simulink model "VsourceInverterZsourceRectifier"  (R2017b)
settings: Solver=ode45  StartTime=0.0  StopTime=0.05  RelTol=1e-3  EnableMultiTasking=on
InitFcn:
  | Fs=100e3;
  | w=Fs*2*pi;
  | 
  | Vdc=100;
  | 
  | LP=200e-6;
  | LS=LP;
  | 
  | CP=1/w^2/LP;
  | CS=1/w^2/LS;
  | 
  | MPS=20e-6;
  | 
  | 
  | Rlp=0.1;
  | Rls=0.1;
libraries: powerlib x30, powerlib_meascontrol x8, simulink x2
settings Model: Creator=User  LastModifiedBy=SuperWindows
settings DataIOCC: FinalStateName=xInitial  LimitDataPoints=on  SaveFinalState=on  SaveFormat=Array
settings OptimizationCC: LifeSpan=inf
settings DebuggingCC: SolverPrmCheckMsg=warning  SFUnexpectedBacktrackingDiag=warning  SFNoUnconditionalDefaultTransitionDiag=warning  SFExecutionAtInitializationDiag=none
settings HardwareCC: ProdBitPerPointer=32  ProdBitPerSizeT=32  ProdBitPerPtrDiffT=32  ProdLargestAtomicFloat=None  ProdIntDivRoundTo=Undefined  ProdEndianess=Unspecified  ProdWordSize=32  ProdHWDeviceType=32-bit Generic
settings ModelReferenceCC: PropagateSignalLabelsOutOfModel=off
settings CodeAppCC: StateflowObjectComments=on
settings GRTTargetCC: TargetLangStandard=C89/C90 (ANSI)  GeneratePreprocessorConditionals=Disable all
settings ConfigComp: CovMetricSettings=dw  CovHtmlReporting=on  CovSaveCumulativeToWorkspaceVar=on  CovSaveSingleToWorkspaceVar=on  CovExternalEMLEnable=off  CovSFcnEnable=off
settings SimscapeCC: SimscapeNormalizeSystem=off

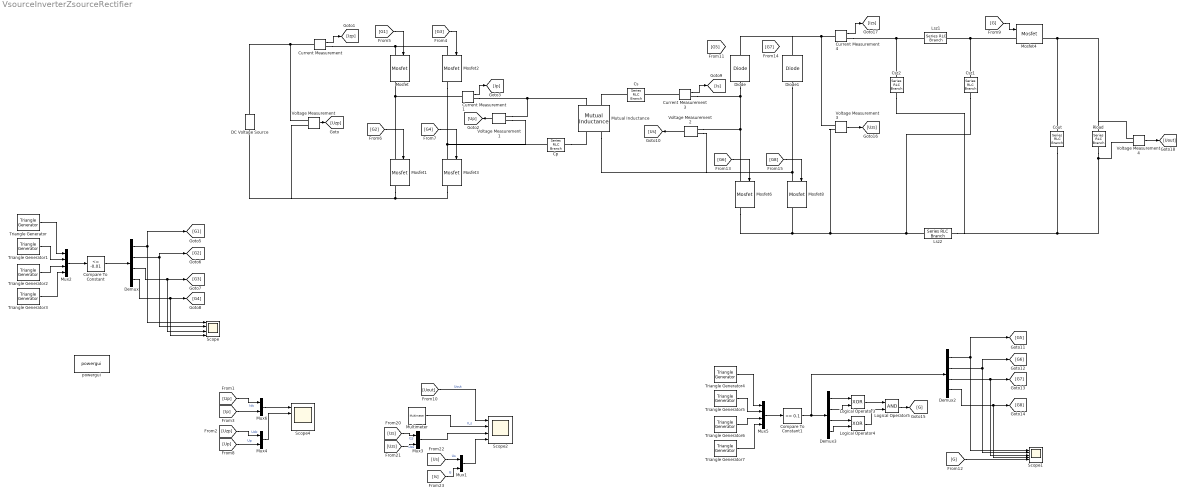
== system VsourceInverterZsourceRectifier ==
  Compare To Constant : simulink/Logic and Bit Operations/Compare To Constant  relop=<=  const=-0.01  OutDataTypeStr=boolean
  Compare To Constant1 : simulink/Logic and Bit Operations/Compare To Constant  relop=<=  const=0.1  OutDataTypeStr=boolean
  Cout : powerlib/Elements/Series RLC Branch  LConnTagsString=__new0  RConnTagsString=__new0  BranchType=C  Resistance=1  Inductance=1e-3  SetiL0=off  InitialCurrent=0  Capacitance=470e-6  Setx0=off  InitialVoltage=100  Measurements=Branch voltage and current
  Cp : powerlib/Elements/Series RLC Branch  LConnTagsString=__new0  RConnTagsString=__new0  BranchType=RC  Resistance=0.02  Inductance=1e-3  SetiL0=off  InitialCurrent=0  Capacitance=13.18e-9  Setx0=off  InitialVoltage=100  Measurements=Branch voltage and current
  Cs : powerlib/Elements/Series RLC Branch  LConnTagsString=__new0  RConnTagsString=__new0  BranchType=RC  Resistance=0.02  Inductance=1e-3  SetiL0=off  InitialCurrent=0  Capacitance=13.42e-9  Setx0=off  InitialVoltage=100  Measurements=Branch voltage and current
  Csz1 : powerlib/Elements/Series RLC Branch  LConnTagsString=__new0  RConnTagsString=__new0  BranchType=C  Resistance=1  Inductance=1e-3  SetiL0=off  InitialCurrent=0  Capacitance=470e-6  Setx0=off  InitialVoltage=100  Measurements=Branch voltage and current
  Csz2 : powerlib/Elements/Series RLC Branch  LConnTagsString=__new0  RConnTagsString=__new0  BranchType=C  Resistance=1  Inductance=1e-3  SetiL0=off  InitialCurrent=0  Capacitance=470e-6  Setx0=off  InitialVoltage=100  Measurements=Branch voltage and current
  Current Measurement{,1,3..4} (4 alike) : powerlib/Measurements/Current Measurement  PhasorSimulation=off  OutputType=Complex  PSBequivalent=0
  DC Voltage Source : powerlib/Electrical Sources/DC Voltage Source  Amplitude=100  Measurements=None
  Demux : Demux
  Demux2 : Demux
  Demux3 : Demux
  Diode : powerlib/Power Electronics/Diode  Ron=0.001  Lon=0  Vf=0.4  IC=0  UseSnubber=0  Rs=inf  Cs=250e-9  Measurements=off
  Diode1 : powerlib/Power Electronics/Diode  Ron=0.001  Lon=0  Vf=0.4  IC=0  UseSnubber=0  Rs=inf  Cs=250e-9  Measurements=off
  Logical Operator3 : Logic  Operator=XOR  AllPortsSameDT=off  OutDataTypeStr=boolean
  Logical Operator4 : Logic  Operator=XOR  AllPortsSameDT=off  OutDataTypeStr=boolean
  Logical Operator5 : Logic  AllPortsSameDT=off  OutDataTypeStr=boolean
  Lsz1 : powerlib/Elements/Series RLC Branch  LConnTagsString=__new0  RConnTagsString=__new0  BranchType=L  Resistance=1  Inductance=1e-3  SetiL0=off  InitialCurrent=0  Capacitance=4700e-6  Setx0=on  InitialVoltage=60  Measurements=Branch voltage and current
  Lsz2 : powerlib/Elements/Series RLC Branch  LConnTagsString=__new0  RConnTagsString=__new0  BranchType=L  Resistance=1  Inductance=1e-3  SetiL0=off  InitialCurrent=0  Capacitance=4700e-6  Setx0=on  InitialVoltage=60  Measurements=Branch voltage and current
  Mosfet{,1..4,6,8} (7 alike) : powerlib/Power Electronics/Mosfet  Ron=0.1  Lon=0  Rd=0.01  Vfd=0  IC=0  Rs=1e5  Cs=inf  Measurements=on
  Multimeter : powerlib/Measurements/Multimeter  PhasorSimulation=off  OutputType=Complex  sel=[14 15]  L=16  Gain=[1 1]  yselected={'Ib: Lsz1','Ib: Lsz2'};  PSBOutputType=1  PSBequivalent=0  AxesSetting=[0,0.1,-100,100]  Display=0  SavedBlockNames=-11
  Mutual Inductance : powerlib/Elements/Mutual Inductance  LConnTagsString=a|b  RConnTagsString=A|B  TypeOfMutual=Two or three windings with equal mutual terms  NumberOfWindings=3  SelfImpedance1=[0.22 263e-06]  SelfImpedance2=[0.22 258e-06]  ThreeWindings=off  SelfImpedance3=[ 1.1 1.1e-03]  MutualImpedance=[0 60e-06]  InductanceMatrix="[1.0 0.9  0.9 ;  0.9 1.0  0.9;  0.9 0.9 1.0 ] * 1e-3"  ResistanceMatrix="[1.0 0.9  0.9 ;  0.9 1.0  0.9;  0.9 0.9 1.0 ]"  Measurements=None
      settings: AttributesFormatString=\n  SourceProductName=Simscape Power Systems  SourceProductBaseCode=PS
  Mux{1,3..4,6} (4 alike) : Mux  Inputs=2
  Mux2 : Mux
  Mux5 : Mux
  Rload : powerlib/Elements/Series RLC Branch  LConnTagsString=__new0  RConnTagsString=__new0  BranchType=R  Resistance=40  Inductance=1e-3  SetiL0=off  InitialCurrent=0  Capacitance=470e-6  Setx0=off  InitialVoltage=100  Measurements=Branch voltage and current
  Scope : Scope  NumInputPorts=4
  Scope1 : Scope  NumInputPorts=5
  Scope2 : Scope  NumInputPorts=4
  Scope4 : Scope  NumInputPorts=4
  Triangle Generator : powerlib_meascontrol/Pulse & Signal Generators/Triangle Generator  Freq=85e3  Phase=0  Ts=0
  Triangle Generator1 : powerlib_meascontrol/Pulse & Signal Generators/Triangle Generator  Freq=85e3  Phase=180  Ts=0
  Triangle Generator2 : powerlib_meascontrol/Pulse & Signal Generators/Triangle Generator  Freq=85e3  Phase=180  Ts=0
  Triangle Generator3 : powerlib_meascontrol/Pulse & Signal Generators/Triangle Generator  Freq=85e3  Phase=0  Ts=0
  Triangle Generator4 : powerlib_meascontrol/Pulse & Signal Generators/Triangle Generator  Freq=85e3  Phase=90  Ts=0
  Triangle Generator5 : powerlib_meascontrol/Pulse & Signal Generators/Triangle Generator  Freq=85e3  Phase=270  Ts=0
  Triangle Generator6 : powerlib_meascontrol/Pulse & Signal Generators/Triangle Generator  Freq=85e3  Phase=270  Ts=0
  Triangle Generator7 : powerlib_meascontrol/Pulse & Signal Generators/Triangle Generator  Freq=85e3  Phase=90  Ts=0
  Voltage Measurement{,1..4} (5 alike) : powerlib/Measurements/Voltage Measurement  PhasorSimulation=off  OutputType=Complex  PSBequivalent=0
  powergui : powerlib/powergui  Priority=1  SimulationMode=Discrete  SampleTime=1e-8  frequency=60  Iterations=50  frequencyindice=0  Pbase=100e6  ErrMax=1e-4  UnitsV=kV  UnitsW=MW  buscounter=0  FunctionMessages=off  echomessages=off  EnableUseOfTLC=off  CurrentSourceSwitches=off  DisableSnubberDevices=off  DisableRonSwitches=off  DisableVfSwitches=off  DisplayEquations=off  SolverType=Tustin/Backward Euler (TBE)  Interpol=off  ExternalGateDelay=off  methode=off  Ts=100  x0status=blocks  SPID=on  SwTol=0  HookPort=off  RestoreLinks=warning  ResistiveCurrentMeasurement=off  Frange=[0:2:500]  Ylog=off  Xlog=on  ShowGrid=off  save=off  variable=ZData  structure=0  ZoomFFT=off  StartTime=0.0  cycles=1  DisplayStyle=1  fundamental=60  FreqAxis=off  MaxFrequency=1000  frequencyindicesteady=1  RmsSteady=1  display=off
  wires:
  Voltage Measurement/1 -> [Uzp]
  Current Measurement/1 -> [Izp]
  Current Measurement1/1 -> [Ip]
  [G1] -> Mosfet/1
  [G4] -> Mosfet3/1
  [G2] -> Mosfet1/1
  [G3] -> Mosfet2/1
  Demux/1 -> [G1], Scope/1
  Demux/2 -> [G2], Scope/2
  Demux/3 -> Scope/3, [G3]
  Demux/4 -> Scope/4, [G4]
  Triangle Generator/1 -> Mux2/1
  Triangle Generator1/1 -> Mux2/2
  Triangle Generator2/1 -> Mux2/3
  Triangle Generator3/1 -> Mux2/4
  Mux2/1 -> Compare To Constant/1
  Compare To Constant/1 -> Demux/1
  Demux3/4 -> Logical Operator4/2
  Compare To Constant1/1 -> Demux2/1, Demux3/1
  Logical Operator3/1 -> Logical Operator5/1
  Logical Operator4/1 -> Logical Operator5/2
  Mux5/1 -> Compare To Constant1/1
  Demux2/4 -> Scope1/4, [G8]
  Triangle Generator5/1 -> Mux5/2
  Demux3/2 -> Logical Operator3/2
  Triangle Generator6/1 -> Mux5/3
  Demux2/1 -> [G5], Scope1/1
  Triangle Generator7/1 -> Mux5/4
  Triangle Generator4/1 -> Mux5/1
  Demux2/3 -> Scope1/3, [G7]
  Demux2/2 -> [G6], Scope1/2
  Demux3/1 -> Logical Operator3/1
  Demux3/3 -> Logical Operator4/1
  Logical Operator5/1 -> [G]
  Voltage Measurement1/1 -> [Up]
  [G] -> Mosfet4/1
  [G6] -> Mosfet6/1
  [G8] -> Mosfet8/1
  [Up] -> Mux4/2  "Up"
  Mux4/1 -> Scope4/2
  Current Measurement3/1 -> [Is]
  Voltage Measurement2/1 -> [Us]
  Voltage Measurement3/1 -> [Uzs]
  Current Measurement4/1 -> [Izs]
  Voltage Measurement4/1 -> [Uout]
  [Uout] -> Scope2/1  "Uout"
  [Is] -> Mux1/2  "Is"
  [Us] -> Mux1/1  "Us"
  Mux1/1 -> Scope2/4
  [G] -> Scope1/5
  [Izs] -> Mux3/1  "Izs"
  [Uzs] -> Mux3/2  "Uzs"
  Mux3/1 -> Scope2/3
  Multimeter/1 -> Scope2/2  "ILs"
  Mux6/1 -> Scope4/1
  [Izp] -> Mux6/1  "Idc"
  [Ip] -> Mux6/2
  [Uzp] -> Mux4/1  "Udc"
  connections:
  Mosfet3/RConn1 -- Voltage Measurement/LConn2 -- DC Voltage Source/LConn1 -- Mosfet1/RConn1
  Current Measurement/LConn1 -- Voltage Measurement/LConn1 -- DC Voltage Source/RConn1
  Mosfet1/LConn1 -- Current Measurement1/LConn1 -- Mosfet/RConn1
  Mosfet2/RConn1 -- Cp/LConn1 -- Voltage Measurement1/LConn2 -- Mosfet3/LConn1
  Mosfet/LConn1 -- Mosfet2/LConn1 -- Current Measurement/RConn1
  Voltage Measurement1/LConn1 -- Current Measurement1/RConn1 -- Mutual Inductance/LConn1
  Cp/RConn1 -- Mutual Inductance/RConn1
  Cs/RConn1 -- Mutual Inductance/LConn2
  Mosfet6/LConn1 -- Diode/LConn1 -- Current Measurement3/RConn1 -- Voltage Measurement2/LConn1
  Mutual Inductance/RConn2 -- Voltage Measurement2/LConn2 -- Diode1/LConn1 -- Mosfet8/LConn1
  Current Measurement4/RConn1 -- Csz2/LConn1 -- Lsz1/RConn1
  Voltage Measurement4/LConn2 -- Csz2/RConn1 -- Lsz2/RConn1 -- Cout/RConn1 -- Rload/RConn1
  Mosfet4/LConn1 -- Lsz1/LConn1 -- Csz1/LConn1
  Cout/LConn1 -- Voltage Measurement4/LConn1 -- Rload/LConn1 -- Mosfet4/RConn1
  Current Measurement3/LConn1 -- Cs/LConn1
  Diode1/RConn1 -- Diode/RConn1 -- Current Measurement4/LConn1 -- Voltage Measurement3/LConn1
  Mosfet6/RConn1 -- Mosfet8/RConn1 -- Voltage Measurement3/LConn2 -- Lsz2/LConn1 -- Csz1/RConn1
